simulink model "FaultDetection_TestHarness"  (R2024b)
settings: Solver=VariableStepAuto  StartTime=0.0  StopTime=+inf  RelTol=1e-3
values from neighbouring files (symbols this model uses):
  CellCurrentLimitThreshold_Fault = 50    [startInit.m]    (also in variables.m)
  CellCurrentLimitThreshold_Warning = 20    [startInit.m]    (also in variables.m)
  CellTemperatureLimitThreshold_Fault = 65    [startInit.m]    (also in variables.m = 338.15)
  CellTemperatureLimitThreshold_Warning = 50    [startInit.m]    (also in variables.m = 323.15)
  CellVoltageLimitHigh_Fault = 4.25    [startInit.m]    (also in variables.m)
  CellVoltageLimitHigh_Warning = 4.21    [startInit.m]    (also in variables.m)
  CellVoltageLimitLow_Fault = 2.65    [startInit.m]    (also in variables.m)
  CellVoltageLimitLow_Warning = 2.70    (= 2.7)    [startInit.m]    (also in variables.m)
libraries: SignalEditorBlockLib x1
settings Model: Creator=E14  LastModifiedBy=E14
settings SolverCC: ZeroCrossAlgorithm=Adaptive
settings DebuggingCC: MaskedZcDiagnostic=none  IgnoredZcDiagnostic=none

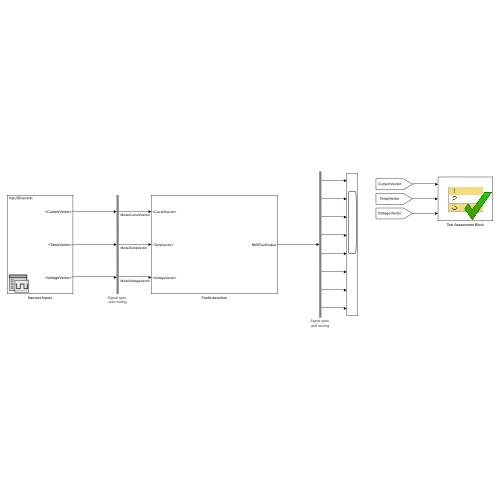
[thumbnail: Simulink's stored preview of the top-level diagram]
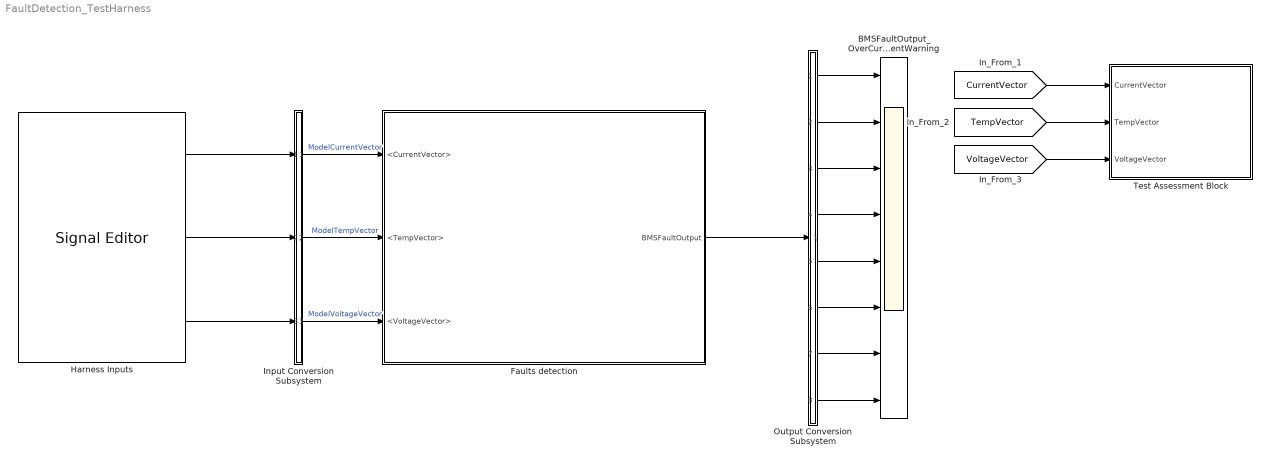
== system FaultDetection_TestHarness ==
  BMSFaultOutput_OverCurrentWarning : Scope
  Faults detection : Subsystem
  Harness Inputs : SignalEditorBlockLib/Signal Editor  FileName=FaultDetection_TestHarness_HarnessInputs.mat  ActiveScenario=InputScenario  ActiveSignal=<VoltageVector>  IsBus=off  OutputBusObjectStr=Bus: BusObject  SampleTime=0.2  Interpolate=off  ZeroCross=off  OutputAfterFinalValue=Setting to zero  Unit=inherit  PreserveSignalName=on  ApplySigPropsToAllScenarios=on  ApplySigPropsToAllSignals=off
  Input Conversion Subsystem : Subsystem  Tag=__SLT_ICS__  Description=|
      | Signal spec.
      | and routing
      settings: AttributesFormatString=%<Description>
  Output Conversion Subsystem : Subsystem  Tag=__SLT_OCS__  Description=|
      | Signal spec.
      | and routing
      settings: AttributesFormatString=%<Description>
  Test Assessment Block : Test Sequence  Tag=__SLT_ASMT__  TreatAsAtomicUnit=on
  wires:
  [CurrentVector] -> Test Assessment Block/1(CurrentVector)
  [TempVector] -> Test Assessment Block/2(TempVector)
  [VoltageVector] -> Test Assessment Block/3(VoltageVector)
  Harness Inputs/1 -> Input Conversion Subsystem/1(Inport_1)
  Harness Inputs/2 -> Input Conversion Subsystem/2(Inport_2)
  Harness Inputs/3 -> Input Conversion Subsystem/3(Inport_3)
  Output Conversion Subsystem/1(Outport_1) -> BMSFaultOutput_OverCurrentWarning/1
  Output Conversion Subsystem/2(Outport_2) -> BMSFaultOutput_OverCurrentWarning/2
  Output Conversion Subsystem/3(Outport_3) -> BMSFaultOutput_OverCurrentWarning/3
  Output Conversion Subsystem/4(Outport_4) -> BMSFaultOutput_OverCurrentWarning/4
  Output Conversion Subsystem/5(Outport_5) -> BMSFaultOutput_OverCurrentWarning/5
  Output Conversion Subsystem/6(Outport_6) -> BMSFaultOutput_OverCurrentWarning/6
  Output Conversion Subsystem/7(Outport_7) -> BMSFaultOutput_OverCurrentWarning/7
  Output Conversion Subsystem/8(Outport_8) -> BMSFaultOutput_OverCurrentWarning/8
  Input Conversion Subsystem/1(Outport_1) -> Faults detection/1(<CurrentVector>)  "ModelCurrentVector"
  Input Conversion Subsystem/2(Outport_2) -> Faults detection/2(<TempVector>)  "ModelTempVector"
  Input Conversion Subsystem/3(Outport_3) -> Faults detection/3(<VoltageVector>)  "ModelVoltageVector"
  Faults detection/1(BMSFaultOutput) -> Output Conversion Subsystem/1(Inport_1)

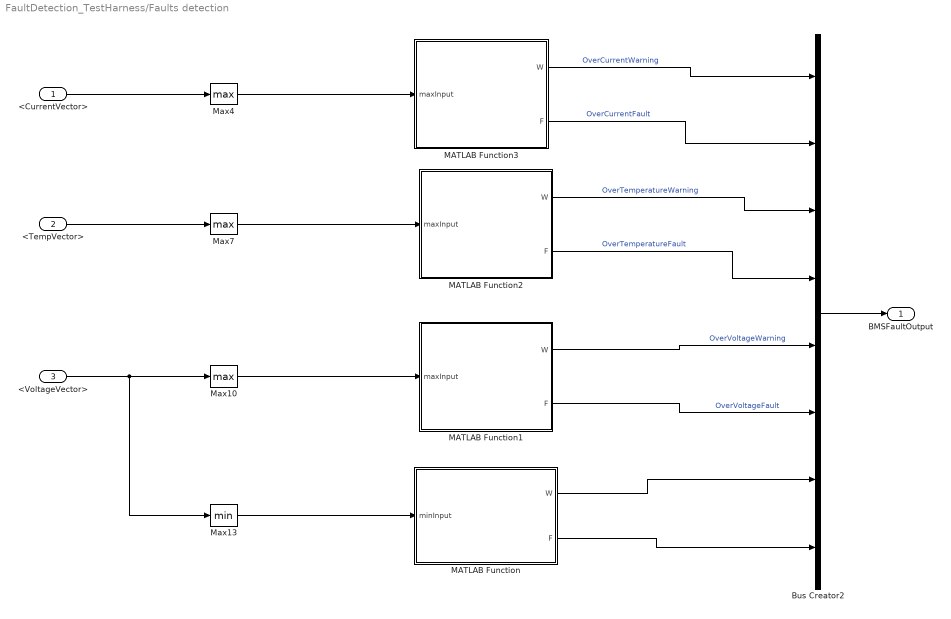
== system FaultDetection_TestHarness/Faults detection ==
  <CurrentVector> : Inport
  <TempVector> : Inport  Port=2
  <VoltageVector> : Inport  Port=3
  Bus Creator2 : BusCreator  Inputs=8
  MATLAB Function : MATLAB Function  TreatAsAtomicUnit=on
  MATLAB Function1 : MATLAB Function  TreatAsAtomicUnit=on
  MATLAB Function2 : MATLAB Function  TreatAsAtomicUnit=on
  MATLAB Function3 : MATLAB Function  TreatAsAtomicUnit=on
  Max10 : MinMax  Function=max
  Max13 : MinMax
  Max4 : MinMax  Function=max
  Max7 : MinMax  Function=max
  BMSFaultOutput : Outport
  wires:
  MATLAB Function2/2(F) -> Bus Creator2/4  "OverTemperatureFault"
  MATLAB Function/2(F) -> Bus Creator2/8
  MATLAB Function/1(W) -> Bus Creator2/7
  Max7/1 -> MATLAB Function2/1(maxInput)
  <VoltageVector>/1 -> Max10/1, Max13/1
  Max10/1 -> MATLAB Function1/1(maxInput)
  <TempVector>/1 -> Max7/1
  MATLAB Function1/1(W) -> Bus Creator2/5  "OverVoltageWarning"
  MATLAB Function1/2(F) -> Bus Creator2/6  "OverVoltageFault"
  Max13/1 -> MATLAB Function/1(minInput)
  MATLAB Function3/2(F) -> Bus Creator2/2  "OverCurrentFault"
  MATLAB Function3/1(W) -> Bus Creator2/1  "OverCurrentWarning"
  <CurrentVector>/1 -> Max4/1
  Max4/1 -> MATLAB Function3/1(maxInput)
  MATLAB Function2/1(W) -> Bus Creator2/3  "OverTemperatureWarning"
  Bus Creator2/1 -> BMSFaultOutput/1

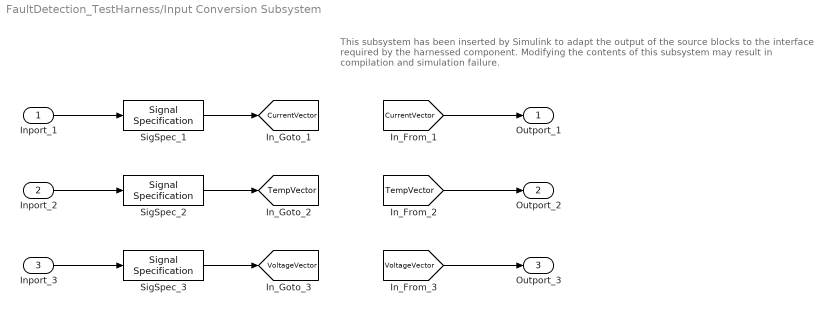
== system FaultDetection_TestHarness/Input Conversion Subsystem ==
  note: This subsystem has been inserted by Simulink to adapt the output of the source blocks to the interface required by the harnessed component.
      |  Modifying the contents of this subsystem may result in compilation and simulation failure.
  Inport_1 : Inport
  Inport_2 : Inport  Port=2
  Inport_3 : Inport  Port=3
  SigSpec_1 : SignalSpecification  OutDataTypeStr=double  Dimensions=[10]  SampleTime=0.2
  SigSpec_2 : SignalSpecification  OutDataTypeStr=double  Dimensions=[10]  SampleTime=0.2
  SigSpec_3 : SignalSpecification  OutDataTypeStr=double  Dimensions=[10]  SampleTime=0.2
  Outport_1 : Outport
  Outport_2 : Outport  Port=2
  Outport_3 : Outport  Port=3
  tag scope: CurrentVector=global, TempVector=global, VoltageVector=global
  wires:
  [CurrentVector] -> Outport_1/1
  SigSpec_1/1 -> [CurrentVector]
  Inport_1/1 -> SigSpec_1/1
  [TempVector] -> Outport_2/1
  SigSpec_2/1 -> [TempVector]
  Inport_2/1 -> SigSpec_2/1
  [VoltageVector] -> Outport_3/1
  SigSpec_3/1 -> [VoltageVector]
  Inport_3/1 -> SigSpec_3/1

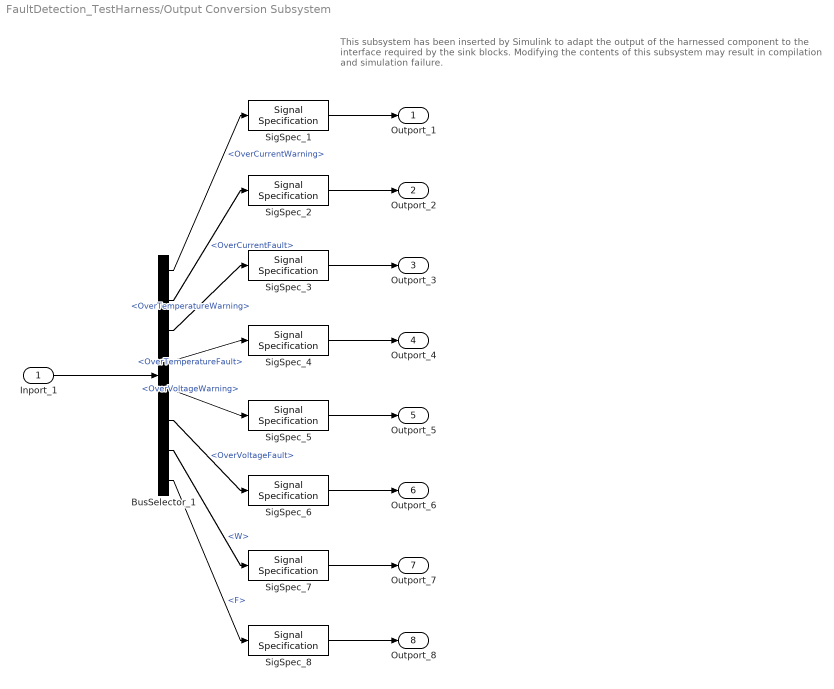
== system FaultDetection_TestHarness/Output Conversion Subsystem ==
  note: This subsystem has been inserted by Simulink to adapt the output of the harnessed component to the interface required by the sink blocks.
      |  Modifying the contents of this subsystem may result in compilation and simulation failure.
  Inport_1 : Inport
  BusSelector_1 : BusSelector  OutputSignals=OverCurrentWarning,OverCurrentFault,OverTemperatureWarning,OverTemperatureFault,OverVoltageWarning,OverVoltageFault,W,F
  SigSpec_{1..8} (8 alike) : SignalSpecification  OutDataTypeStr=double  Dimensions=[1]  SampleTime=0.2
  Outport_1 : Outport
  Outport_2 : Outport  Port=2
  Outport_3 : Outport  Port=3
  Outport_4 : Outport  Port=4
  Outport_5 : Outport  Port=5
  Outport_6 : Outport  Port=6
  Outport_7 : Outport  Port=7
  Outport_8 : Outport  Port=8
  wires:
  Inport_1/1 -> BusSelector_1/1
  BusSelector_1/1 -> SigSpec_1/1  "<OverCurrentWarning>"
  SigSpec_1/1 -> Outport_1/1
  BusSelector_1/2 -> SigSpec_2/1  "<OverCurrentFault>"
  SigSpec_2/1 -> Outport_2/1
  BusSelector_1/3 -> SigSpec_3/1  "<OverTemperatureWarning>"
  SigSpec_3/1 -> Outport_3/1
  BusSelector_1/4 -> SigSpec_4/1  "<OverTemperatureFault>"
  SigSpec_4/1 -> Outport_4/1
  BusSelector_1/5 -> SigSpec_5/1  "<OverVoltageWarning>"
  SigSpec_5/1 -> Outport_5/1
  BusSelector_1/6 -> SigSpec_6/1  "<OverVoltageFault>"
  SigSpec_6/1 -> Outport_6/1
  BusSelector_1/7 -> SigSpec_7/1  "<W>"
  SigSpec_7/1 -> Outport_7/1
  BusSelector_1/8 -> SigSpec_8/1  "<F>"
  SigSpec_8/1 -> Outport_8/1

== matlab function FaultDetection_TestHarness/Faults detection/MATLAB Function3 ==
  data: maxInput input; W output; F output; CellCurrentLimitThreshold_Warning parameter; CellCurrentLimitThreshold_Fault parameter
function [W, F] = overCurrent( maxInput,CellCurrentLimitThreshold_Warning, CellCurrentLimitThreshold_Fault)
W=0;
F=0;
if maxInput >= CellCurrentLimitThreshold_Warning && maxInput < CellCurrentLimitThreshold_Fault

    W=1;
    F=0;
elseif maxInput >= CellCurrentLimitThreshold_Fault
    W=0;
    F=1;
end

end

== stateflow chart FaultDetection_TestHarness/Test Assessment Block ==
  state Run
    state step_1_1
    state step_1_2
    (default) -> (junction 22)
    Run -> (junction 22)
    (junction 22) -> (junction 23) [order 1] : [t < 5
        | ]
    (junction 23) -> step_1_1 [order 1] : [~in(Run.step_1_1)]
    (junction 23) -> (junction 26) [order 2]
    (junction 31) -> (junction 32)
    (junction 32) -> step_1_2 [order 1] : [~in(Run.step_1_2)]
    (junction 32) -> (junction 35) [order 2]
    (junction 22) -> (junction 31) [order 2]
  (default) -> Run
  data: CurrentVector input double size=[10]; TempVector input double size=[10]; VoltageVector input double size=[10]

== matlab function FaultDetection_TestHarness/Faults detection/MATLAB Function ==
  data: minInput input; W output; F output; CellVoltageLimitLow_Warning parameter; CellVoltageLimitLow_Fault parameter
function [W,F] = underVoltage(minInput,CellVoltageLimitLow_Warning, CellVoltageLimitLow_Fault)
W=0;
F=0;
if minInput <= CellVoltageLimitLow_Warning && minInput > CellVoltageLimitLow_Fault
    W=1;
    F=0;
elseif minInput <= CellVoltageLimitLow_Fault
    W=0;
    F=1;
end
end

== matlab function FaultDetection_TestHarness/Faults detection/MATLAB Function1 ==
  data: maxInput input; W output; F output; CellVoltageLimitHigh_Warning parameter; CellVoltageLimitHigh_Fault parameter
function [W, F] = overVoltage( maxInput,CellVoltageLimitHigh_Warning, CellVoltageLimitHigh_Fault)
W=0;
F=0;
if maxInput >= CellVoltageLimitHigh_Warning && maxInput < CellVoltageLimitHigh_Fault

    W=1;
    F=0;
elseif maxInput >= CellVoltageLimitHigh_Fault
    W=0;
    F=1;
end

end

== matlab function FaultDetection_TestHarness/Faults detection/MATLAB Function2 ==
  data: maxInput input; W output; F output; CellTemperatureLimitThreshold_Warning parameter; CellTemperatureLimitThreshold_Fault parameter
function [W, F] = tempreture( maxInput,CellTemperatureLimitThreshold_Warning, CellTemperatureLimitThreshold_Fault)
W=0;
F=0;
if maxInput >= CellTemperatureLimitThreshold_Warning && maxInput < CellTemperatureLimitThreshold_Fault

    W=1;
    F=0;
elseif maxInput >= CellTemperatureLimitThreshold_Fault
    W=0;
    F=1;
end

end
